simulink model "rv2Sim"  (R2022b)
settings: Solver=FixedStepAuto  StartTime=0.0  StopTime=86400  FixedStep=1  RelTol=1e-3
undefined symbols (not defined in the file or in its folder): modes, rv2
settings Model: SimulationMode=accelerator  Creator=HelloWorld  LastModifiedBy=HelloWorld

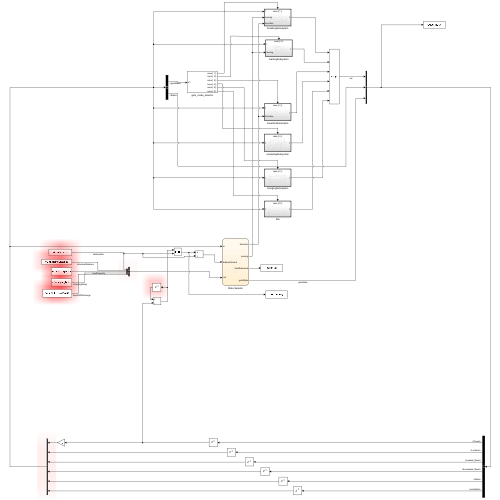
[thumbnail: Simulink's stored preview of the top-level diagram]
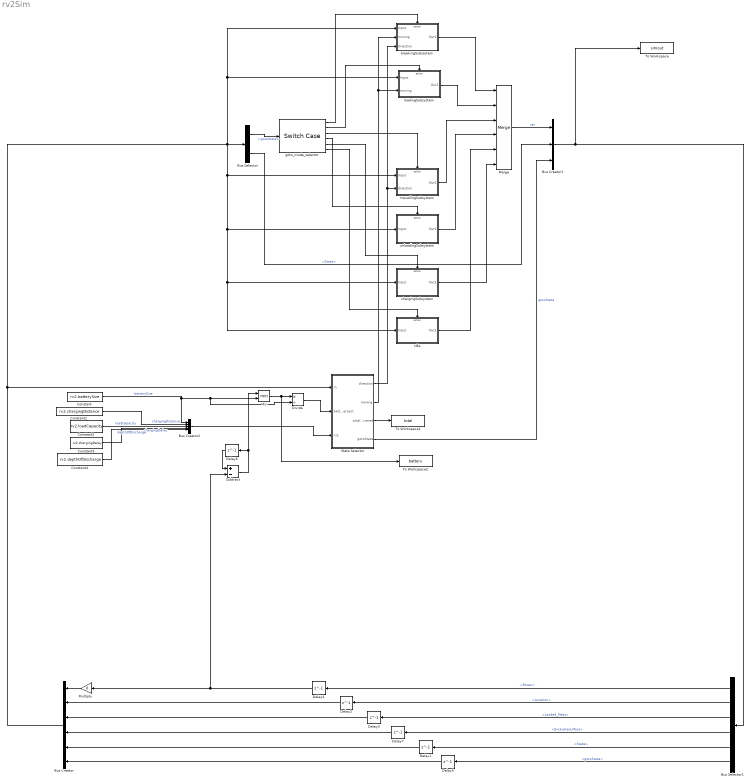
== system rv2Sim ==
  Bus Creator : BusCreator  Inputs=6  OutDataTypeStr=Bus: curState
      settings: InheritFromInputs=off
  Bus Creator1 : BusCreator  Inputs=3
  Bus Creator2 : BusCreator  Inputs=5  OutDataTypeStr=Bus: bus_rv
  Bus Selector : BusSelector  OutputSignals=gotoState,State
  Bus Selector1 : BusSelector  OutputSignals=var.Power,var.Location,var.Loaded_Mass,var.Excavated_Mass,State,gotoState
  Constant : Constant  Value=rv2.batterySize
  Constant1 : Constant  Value=rv2.chargingDistance
  Constant2 : Constant  Value=rv2.loadCapacity
  Constant3 : Constant  Value=rv2.chargingDelay
  Constant4 : Constant  Value=rv2.depthOfDischarge
  Delay1 : Delay  DelayLength=1  InitialCondition=int8(modes.breaking)
  Delay{2..4,7} (4 alike) : Delay  DelayLength=1  InitialCondition=0
  Delay5 : Delay  DelayLength=1  InitialCondition=int8(modes.idle)
  Delay6 : Delay  DelayLength=1  InitialCondition=rv2.batterySize
  Divide : Product  Inputs=*/
  Idle : Subsystem  TreatAsAtomicUnit=on
  Merge : Merge  Inputs=6
  Min : MinMax  Inputs=2
  Multiply : Gain  Gain=0
  State Selector : Stateflow chart  TreatAsAtomicUnit=on
  Subtract : Sum  Inputs=+-
  To Workspace : ToWorkspace  VariableName=simout  SaveFormat=Timeseries  SampleTime=-1
  To Workspace1 : ToWorkspace  VariableName=total  SampleTime=-1
      settings: Save2DSignal=2-D array (concatenate along first dimension)
  To Workspace2 : ToWorkspace  VariableName=battery  SampleTime=-1
      settings: Save2DSignal=2-D array (concatenate along first dimension)
  breakingSubssytem : Subsystem  TreatAsAtomicUnit=on
  chargingSubsystem : Subsystem  TreatAsAtomicUnit=on
  goto_mode_selector : SwitchCase  CaseConditions={1, 2, 3, 4, 5, 0}  ShowDefaultCase=off
  loadingSubsystem : Subsystem  TreatAsAtomicUnit=on
  travellingSubsystem : Subsystem  TreatAsAtomicUnit=on
  unloadingSubsystem : Subsystem  TreatAsAtomicUnit=on
  wires:
  goto_mode_selector/1 -> breakingSubssytem/Action
  goto_mode_selector/2 -> loadingSubsystem/Action
  goto_mode_selector/3 -> travellingSubsystem/Action
  breakingSubssytem/1(Out1) -> Merge/1
  loadingSubsystem/1(Out1) -> Merge/2
  travellingSubsystem/1(Out1) -> Merge/3
  Bus Selector/1 -> goto_mode_selector/1  "<gotoState>"
  Bus Selector1/1 -> Delay4/1  "<Power>"
  Bus Selector1/2 -> Delay2/1  "<Location>"
  Bus Selector1/3 -> Delay3/1  "<Loaded_Mass>"
  Bus Selector1/5 -> Delay1/1  "<State>"
  Bus Selector1/6 -> Delay5/1  "<gotoState>"
  Bus Creator/1 -> breakingSubssytem/1(Input), loadingSubsystem/1(Input), Idle/1(Input), chargingSubsystem/1(Input), unloadingSubsystem/1(Input), travellingSubsystem/1(Input), Bus Selector/1, State Selector/1(in)
  Delay1/1 -> Bus Creator/5
  Delay2/1 -> Bus Creator/2
  Delay3/1 -> Bus Creator/3
  Delay4/1 -> Multiply/1, Subtract/2
  Delay5/1 -> Bus Creator/6
  Multiply/1 -> Bus Creator/1
  Bus Creator1/1 -> To Workspace/1, Bus Selector1/1
  Merge/1 -> Bus Creator1/1  "var"
  Bus Selector/2 -> Bus Creator1/2  "<State>"
  State Selector/4(gotoState) -> Bus Creator1/3  "gotoState"
  State Selector/1(direction) -> breakingSubssytem/3(direction), travellingSubsystem/2(direction)
  goto_mode_selector/4 -> unloadingSubsystem/Action
  unloadingSubsystem/1(Out1) -> Merge/4
  Idle/1(Out1) -> Merge/5
  State Selector/3(totalDelivered) -> To Workspace1/1
  goto_mode_selector/5 -> chargingSubsystem/Action
  goto_mode_selector/6 -> Idle/Action
  chargingSubsystem/1(Out1) -> Merge/6
  Subtract/1 -> Min/1, Delay6/1
  Delay6/1 -> Subtract/1
  Min/1 -> To Workspace2/1, Divide/1
  Bus Selector1/4 -> Delay7/1  "<Excavated_Mass>"
  Delay7/1 -> Bus Creator/4
  Constant/1 -> Divide/2, Min/2, Bus Creator2/1  "batterySize"
  Constant1/1 -> Bus Creator2/2  "chargingDistance"
  Constant2/1 -> Bus Creator2/3  "loadCapacity"
  Bus Creator2/1 -> State Selector/3(rv2)
  Divide/1 -> State Selector/2(batteryPercent)
  State Selector/2(moving) -> breakingSubssytem/2(moving), loadingSubsystem/2(moving)
  Constant3/1 -> Bus Creator2/4  "chargingDelay"
  Constant4/1 -> Bus Creator2/5  "depthOfDischarge"

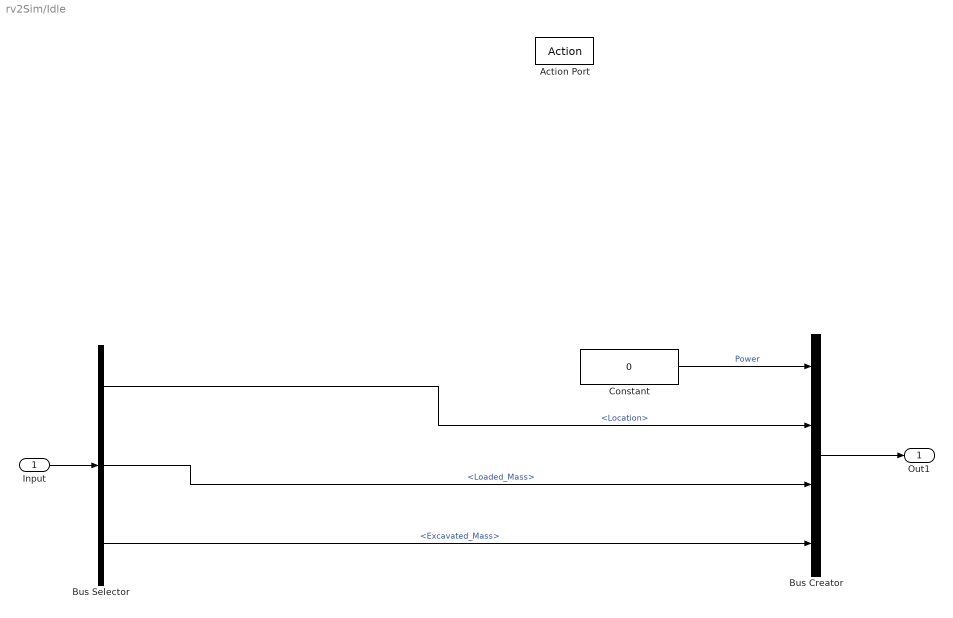
== system rv2Sim/Idle ==
  Input : Inport  OutDataTypeStr=Bus: curState
  Action Port : ActionPort  ActionPortLabel=case [ 0 ]:
  Bus Creator : BusCreator  Inputs=4
  Bus Selector : BusSelector  OutputSignals=Location,Loaded_Mass,Excavated_Mass
  Constant : Constant  Value=0
  Out1 : Outport  LockScale=on
  wires:
  Input/1 -> Bus Selector/1
  Constant/1 -> Bus Creator/1  "Power"
  Bus Creator/1 -> Out1/1
  Bus Selector/3 -> Bus Creator/4  "<Excavated_Mass>"
  Bus Selector/2 -> Bus Creator/3  "<Loaded_Mass>"
  Bus Selector/1 -> Bus Creator/2  "<Location>"

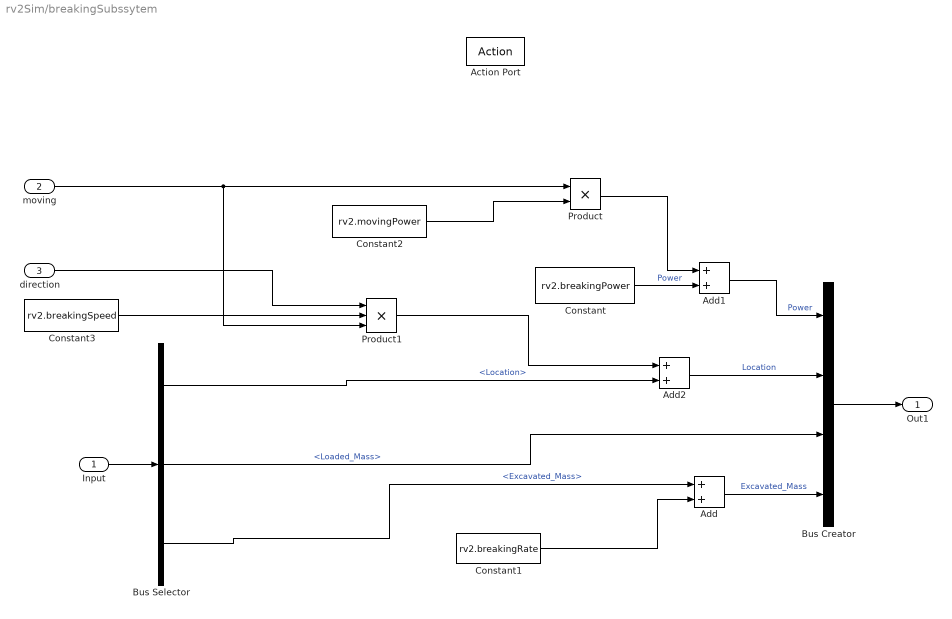
== system rv2Sim/breakingSubssytem ==
  Input : Inport  OutDataTypeStr=Bus: curState
  moving : Inport  Port=2
  direction : Inport  Port=3
  Action Port : ActionPort  ActionPortLabel=case [ 1 ]:
  Add : Sum
  Add1 : Sum
  Add2 : Sum
  Bus Creator : BusCreator  Inputs=4
  Bus Selector : BusSelector  OutputSignals=Location,Loaded_Mass,Excavated_Mass
  Constant : Constant  Value=rv2.breakingPower
  Constant1 : Constant  Value=rv2.breakingRate
  Constant2 : Constant  Value=rv2.movingPower
  Constant3 : Constant  Value=rv2.breakingSpeed
  Product : Product
  Product1 : Product  Inputs=3
  Out1 : Outport  LockScale=on
  wires:
  Input/1 -> Bus Selector/1
  Constant1/1 -> Add/2
  Add1/1 -> Bus Creator/1  "Power"
  Bus Selector/2 -> Bus Creator/3  "<Loaded_Mass>"
  Bus Selector/3 -> Add/1  "<Excavated_Mass>"
  Add/1 -> Bus Creator/4  "Excavated_Mass"
  Bus Creator/1 -> Out1/1
  moving/1 -> Product1/3, Product/1
  Constant2/1 -> Product/2
  Product/1 -> Add1/1
  Constant/1 -> Add1/2  "Power"
  Constant3/1 -> Product1/2
  Product1/1 -> Add2/1
  Bus Selector/1 -> Add2/2  "<Location>"
  Add2/1 -> Bus Creator/2  "Location"
  direction/1 -> Product1/1

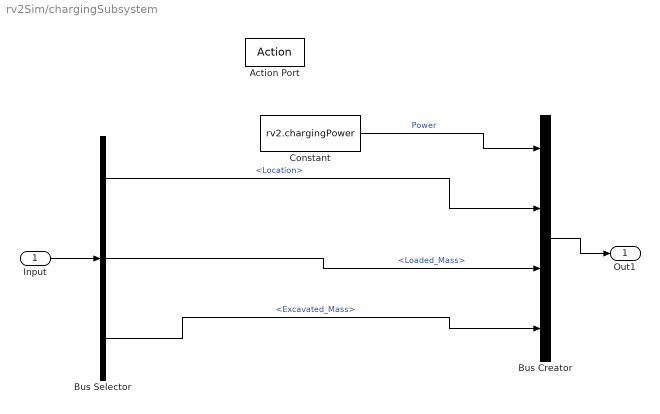
== system rv2Sim/chargingSubsystem ==
  Input : Inport  OutDataTypeStr=Bus: curState
  Action Port : ActionPort  ActionPortLabel=case [ 5 ]:
  Bus Creator : BusCreator  Inputs=4
  Bus Selector : BusSelector  OutputSignals=Location,Loaded_Mass,Excavated_Mass
  Constant : Constant  Value=rv2.chargingPower
  Out1 : Outport  LockScale=on
  wires:
  Input/1 -> Bus Selector/1
  Constant/1 -> Bus Creator/1  "Power"
  Bus Selector/1 -> Bus Creator/2  "<Location>"
  Bus Creator/1 -> Out1/1
  Bus Selector/3 -> Bus Creator/4  "<Excavated_Mass>"
  Bus Selector/2 -> Bus Creator/3  "<Loaded_Mass>"

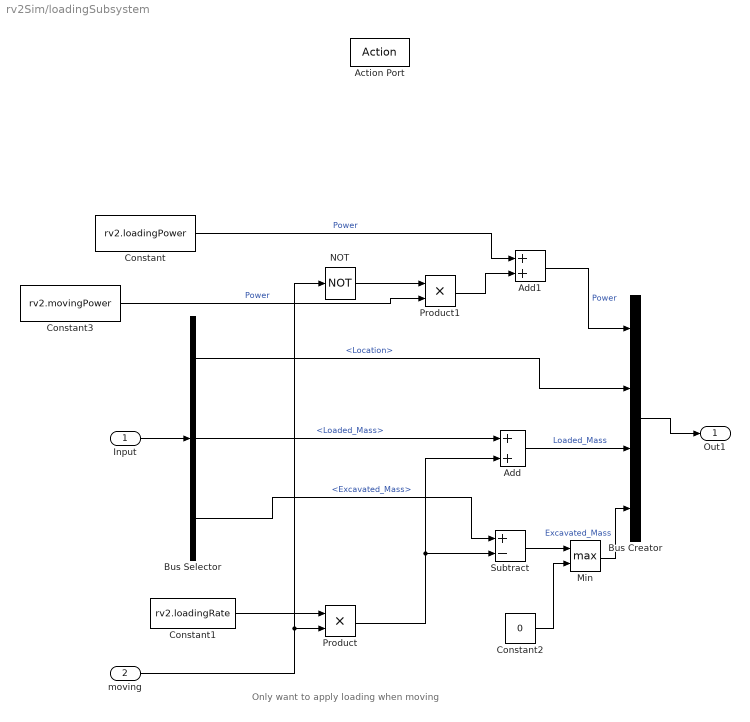
== system rv2Sim/loadingSubsystem ==
  note: Only want to apply loading when moving
  Input : Inport  OutDataTypeStr=Bus: curState
  moving : Inport  Port=2
  Action Port : ActionPort  ActionPortLabel=case [ 2 ]:
  Add : Sum
  Add1 : Sum
  Bus Creator : BusCreator  Inputs=4
  Bus Selector : BusSelector  OutputSignals=Location,Loaded_Mass,Excavated_Mass
  Constant : Constant  Value=rv2.loadingPower
  Constant1 : Constant  Value=rv2.loadingRate
  Constant2 : Constant  Value=0
  Constant3 : Constant  Value=rv2.movingPower
  Min : MinMax  Function=max  Inputs=2
  NOT : Logic  Operator=NOT  IconShape=distinctive  AllPortsSameDT=off  OutDataTypeStr=boolean
  Product : Product
  Product1 : Product
  Subtract : Sum  Inputs=+-
  Out1 : Outport  LockScale=on
  wires:
  Input/1 -> Bus Selector/1
  Constant/1 -> Add1/1  "Power"
  Bus Selector/1 -> Bus Creator/2  "<Location>"
  Bus Creator/1 -> Out1/1
  Add/1 -> Bus Creator/3  "Loaded_Mass"
  Bus Selector/2 -> Add/1  "<Loaded_Mass>"
  Bus Selector/3 -> Subtract/1  "<Excavated_Mass>"
  Subtract/1 -> Min/1
  Min/1 -> Bus Creator/4  "Excavated_Mass"
  Constant2/1 -> Min/2
  Constant1/1 -> Product/1
  moving/1 -> NOT/1, Product/2
  Product/1 -> Add/2, Subtract/2
  NOT/1 -> Product1/1
  Constant3/1 -> Product1/2  "Power"
  Product1/1 -> Add1/2
  Add1/1 -> Bus Creator/1  "Power"

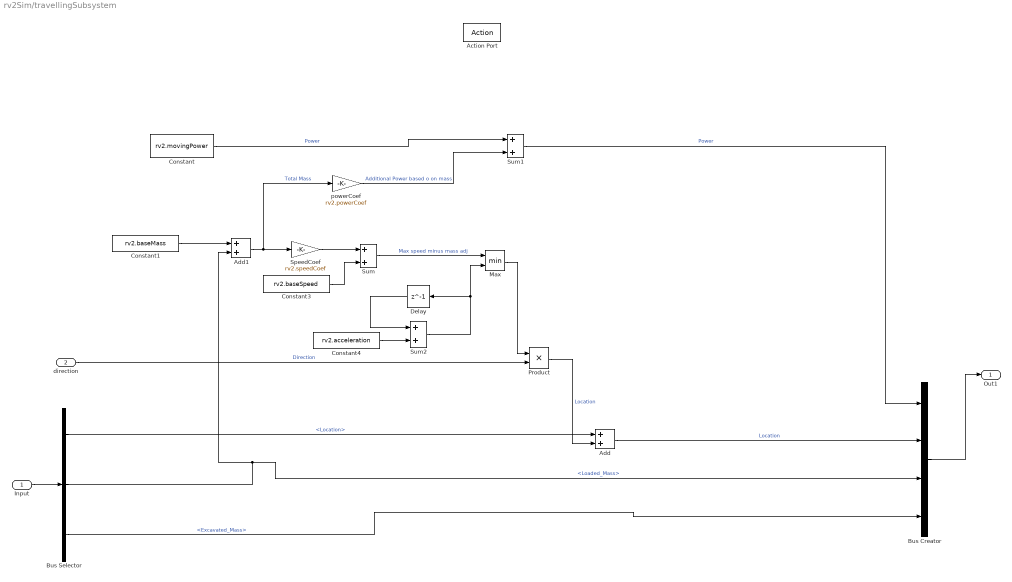
== system rv2Sim/travellingSubsystem ==
  Input : Inport  OutDataTypeStr=Bus: curState
  direction : Inport  Port=2
  Action Port : ActionPort  InitializeStates=reset  ActionPortLabel=case [ 3 ]:
  Add : Sum
  Add1 : Sum
  Bus Creator : BusCreator  Inputs=4
  Bus Selector : BusSelector  OutputSignals=Location,Loaded_Mass,Excavated_Mass
  Constant : Constant  Value=rv2.movingPower
  Constant1 : Constant  Value=rv2.baseMass
  Constant3 : Constant  Value=rv2.baseSpeed
  Constant4 : Constant  Value=rv2.acceleration
  Delay : Delay  DelayLength=1
  Max : MinMax  Inputs=2
  Product : Product
  SpeedCoef : Gain  Gain=rv2.speedCoef
  Sum : Sum
  Sum1 : Sum
  Sum2 : Sum
  powerCoef : Gain  Gain=rv2.powerCoef
  Out1 : Outport  LockScale=on
  wires:
  Input/1 -> Bus Selector/1
  Bus Creator/1 -> Out1/1
  Constant1/1 -> Add1/1
  Add1/1 -> powerCoef/1, SpeedCoef/1  "Total Mass"
  SpeedCoef/1 -> Sum/1
  Bus Selector/1 -> Add/1  "<Location>"
  Bus Selector/3 -> Bus Creator/4  "<Excavated_Mass>"
  Bus Selector/2 -> Bus Creator/3, Add1/2  "<Loaded_Mass>"
  Product/1 -> Add/2  "Location"
  Add/1 -> Bus Creator/2  "Location"
  direction/1 -> Product/2  "Direction"
  powerCoef/1 -> Sum1/2  "Additional Power based o on mass"
  Constant/1 -> Sum1/1  "Power"
  Sum1/1 -> Bus Creator/1  "Power"
  Sum/1 -> Max/1  "Max speed minus mass adj"
  Constant3/1 -> Sum/2
  Constant4/1 -> Sum2/2
  Sum2/1 -> Delay/1, Max/2
  Delay/1 -> Sum2/1
  Max/1 -> Product/1

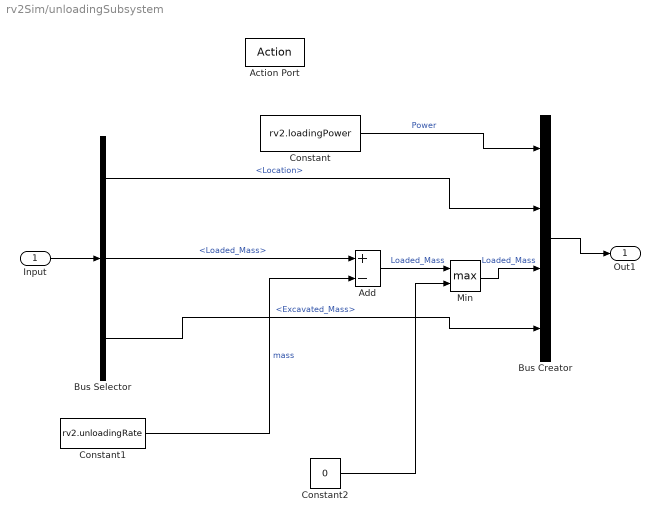
== system rv2Sim/unloadingSubsystem ==
  Input : Inport  OutDataTypeStr=Bus: curState
  Action Port : ActionPort  ActionPortLabel=case [ 4 ]:
  Add : Sum  Inputs=+-
  Bus Creator : BusCreator  Inputs=4
  Bus Selector : BusSelector  OutputSignals=Location,Loaded_Mass,Excavated_Mass
  Constant : Constant  Value=rv2.loadingPower
  Constant1 : Constant  Value=rv2.unloadingRate
  Constant2 : Constant  Value=0
  Min : MinMax  Function=max  Inputs=2
  Out1 : Outport  LockScale=on
  wires:
  Input/1 -> Bus Selector/1
  Constant/1 -> Bus Creator/1  "Power"
  Bus Selector/1 -> Bus Creator/2  "<Location>"
  Bus Creator/1 -> Out1/1
  Bus Selector/2 -> Add/1  "<Loaded_Mass>"
  Bus Selector/3 -> Bus Creator/4  "<Excavated_Mass>"
  Constant1/1 -> Add/2  "mass"
  Constant2/1 -> Min/2
  Add/1 -> Min/1  "Loaded_Mass"
  Min/1 -> Bus Creator/3  "Loaded_Mass"

== stateflow chart rv2Sim/State Selector ==
  state Done
    gotoState=int8(modes.idle);
  state Init
    gotoState=int8(modes.idle);
    direction=1;
    totalDelivered=0;
    load=0;
    moving=0;
    state=0;
    cycle_count=0;
  state Idle
    gotoState=int8(modes.idle);
  state Charging
    du:
    gotoState=int8(modes.charging);
  state Excavate
    gotoState=int8(modes.breaking);
    state startJackhammer
      du:
      moving=0;
      direction=1;
    state moveForward
      du:
      moving=1;
      direction=direction*-1;
    state stopMoving
      du:
      moving=0;
    (default) -> startJackhammer
    startJackhammer -> moveForward : after(5,tick)
    moveForward -> stopMoving : after(20, sec)
  state MoveToPit
    entry:
    cycle_count=cycle_count+1;
    du:
    gotoState=int8(modes.travelling);
    direction=-1;
  state Load
    gotoState=int8(modes.loading);
    state lowerScoop
      du:
      moving=0;
    state adjustScoop
      du:
      moving=0;
    state move
      du:
      moving=1;
      direction=direction*-1;
    (default) -> lowerScoop
    lowerScoop -> move : after(10, sec)
    move -> adjustScoop : after(20, sec)
  state Unload
    gotoState=int8(modes.unloading);
  state MoveToSite
    gotoState=int8(modes.travelling);
    direction=1;
    load=in.Loaded_Mass;
  Charging -> Done [order 2] : [totalDelivered>400 & batteryPercent>0.99]
  (default) -> Init
  Init -> Idle
  Idle -> Excavate : [in.Excavated_Mass <= rv2.loadCapacity]
  Excavate -> (junction 113) : [totalDelivered>400]
  (junction 113) -> Charging : after(rv2.chargingDelay, sec)
  Charging -> Excavate [order 1] : [batteryPercent>0.99 & totalDelivered<400]
  stopMoving -> (junction 79) : after(60, sec)
  (junction 90) -> Charging : after(rv2.chargingDelay, sec)
  (junction 115) -> Charging [order 1] : [cycle_count==2]
  (junction 79) -> moveForward [order 2] : [in.Excavated_Mass<rv2.loadCapacity]
  (junction 62) -> (junction 90) [order 2] : [batteryPercent < rv2.depthOfDischarge]
      | {gotoState=int8(modes.idle)}
  (junction 115) -> Excavate [order 2]
  (junction 79) -> (junction 62) [order 1] : [in.Excavated_Mass >= rv2.loadCapacity]
  MoveToPit -> (junction 115) : [in.Location <=0.1]
  (junction 62) -> Load [order 1] : [batteryPercent>=rv2.depthOfDischarge]
  Unload -> MoveToPit : [in.Loaded_Mass <=0]
      | {totalDelivered=totalDelivered+load;}
  (junction 104) -> lowerScoop [order 2] : [in.Loaded_Mass <rv2.loadCapacity]
  adjustScoop -> (junction 104) : after(10, sec)
  MoveToSite -> Unload : [in.Location >= 500]
  (junction 104) -> MoveToSite [order 1] : [in.Loaded_Mass >= rv2.loadCapacity]
  data: direction output; moving output; totalDelivered output double; in input Bus: curState; batteryPercent input; gotoState output int8; load local; rv2 input; state local; cycle_count local
